simulink library "EOIRParametricModelBlock"  (R2018b)
settings: Solver=VariableStepAuto  StartTime=0.0  StopTime=10.0  RelTol=1e-3
undefined symbols (not defined in the file): ac1dyn_alt0_ft, ac1dyn_lat0_rad, ac1dyn_lon0_rad, ac1IntEOIR_az_bias_rad, ac1IntEOIR_az_random_stddev_rad, ac1IntEOIR_az_tau_s, ac1IntEOIR_azdot_bias_radps, ac1IntEOIR_azdot_random_stddev_radps, ac1IntEOIR_azdot_tau_s, ac1IntEOIR_dt_s, ac1IntEOIR_el_bias_rad, ac1IntEOIR_el_random_stddev_rad, ac1IntEOIR_el_tau_s, ac1IntEOIR_eldot_bias_radps, ac1IntEOIR_eldot_random_stddev_radps, ac1IntEOIR_eldot_tau_s, ac1IntEOIR_range_clrd_noise_flag, ac1IntEOIR_reported_errorCovRAE, ac1IntEOIR_rng_bias_ft, ac1IntEOIR_rng_bias_switch, ac1IntEOIR_rng_random_stddev_ft, ac1IntEOIR_rng_std_dev_gain, ac1IntEOIR_rng_tau_s, ac1IntEOIR_rngdot_bias_ftps, ac1IntEOIR_rngdot_delay_s, ac1IntEOIR_rngdot_random_stddev_ftps, ac1IntEOIR_rngdot_std_dev_gain, ac1IntEOIR_rngdot_tau_s, ac1IntEOIR_seed1, ac1IntEOIR_seed2, ac1IntEOIR_seed3, ac1IntEOIR_seed4, ac1IntEOIR_seed5, ac1IntEOIR_seed6, ac1IntEOIR_sns_for_azimuth_deg, ac1IntEOIR_sns_for_elevation_deg, ac1IntEOIR_sns_max_range_ft
libraries: simulink x11, cart2sph_degas x1, ExtractCovDiag x1, sph2cart x1
settings Model: Creator=BI28030  LastModifiedBy=BI28030
settings SFSimCC: SimUseLocalCustomCode=off
settings RTWCC: RTWUseLocalCustomCode=off
settings CodeAppCC: StateflowObjectComments=on

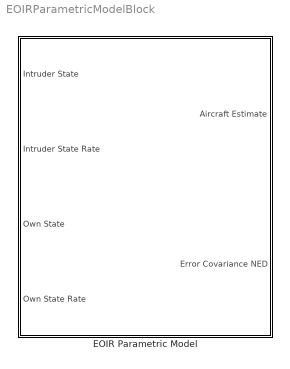
== system EOIRParametricModelBlock ==
  EOIR Parametric Model : Subsystem  mask(EOIR Parametric Model){dt_s=ac1IntEOIR_dt_s, lat0_rad=ac1dyn_lat0_rad, lon0_rad=ac1dyn_lon0_rad, alt0_ft=ac1dyn_alt0_ft, sns_max_range_ft=ac1IntEOIR_sns_max_range_ft, sns_for_azimuth_deg=ac1IntEOIR_sns_for_azimuth_deg, sns_for_elevation_deg=ac1IntEOIR_sns_for_elevation_deg, rng_random_stddev_ft=ac1IntEOIR_rng_random_stddev_ft, rng_bias_ft=ac1IntEOIR_rng_bias_ft, rng_tau_s=ac1IntEOIR_rng_tau_s, seed1=ac1IntEOIR_seed1, rng_std_dev_gain=ac1IntEOIR_rng_std_dev_gain, rng_bias_switch=ac1IntEOIR_rng_bias_switch, coloredNoiseFlag=ac1IntEOIR_range_clrd_noise_flag, az_random_stddev_rad=ac1IntEOIR_az_random_stddev_rad, az_bias_rad=ac1IntEOIR_az_bias_rad, az_tau_s=ac1IntEOIR_az_tau_s, seed2=ac1IntEOIR_seed2, el_random_stddev_rad=ac1IntEOIR_el_random_stddev_rad, el_bias_rad=ac1IntEOIR_el_bias_rad, el_tau_s=ac1IntEOIR_el_tau_s, seed3=ac1IntEOIR_seed3, rngdot_random_stddev_ftps=ac1IntEOIR_rngdot_random_stddev_ftps, rngdot_bias_ftps=ac1IntEOIR_rngdot_bias_ftps, rngdot_tau_s=ac1IntEOIR_rngdot_tau_s, seed4=ac1IntEOIR_seed4, rngdot_std_dev_gain=ac1IntEOIR_rngdot_std_dev_gain, rngdot_delay_s=ac1IntEOIR_rngdot_delay_s, azdot_random_stddev_radps=ac1IntEOIR_azdot_random_stddev_radps, azdot_bias_radps=ac1IntEOIR_azdot_bias_radps, azdot_tau_s=ac1IntEOIR_azdot_tau_s, seed5=ac1IntEOIR_seed5, eldot_random_stddev_radps=ac1IntEOIR_eldot_random_stddev_radps, eldot_bias_radps=ac1IntEOIR_eldot_bias_radps, eldot_tau_s=ac1IntEOIR_eldot_tau_s, seed6=ac1IntEOIR_seed6, covRAE=ac1IntEOIR_reported_errorCovRAE}
      mask prompts: dt_s "Timestep"; lat0_rad "ENU Origin Latitude"; lon0_rad "ENU Origin Longitude"; alt0_ft "ENU Origin Altitude"; sns_max_range_ft "Max Detection Range"; sns_for_azimuth_deg "Field of Regard: Azimuth Limit (deg)"; sns_for_elevation_deg "Field of Regard: Elevation Limit (deg)"; rng_random_stddev_ft "Range Random Error Standard Deviation"; rng_bias_ft "Range Bias"; rng_tau_s "Correlation Time"; seed1 "Random Seed"; rng_std_dev_gain "Standard Deviation gain"; rng_bias_switch "Range Bias Switch"; coloredNoiseFlag "Range Colored Noise Switch"; az_random_stddev_rad "Azimuth Random Error Standard Deviation"; az_bias_rad "Azimuth Bias"; az_tau_s "Correlation Time"; seed2 "Random Seed"; el_random_stddev_rad "Elevation Random Error Standard Deviation"; el_bias_rad "Elevation Bias"; el_tau_s "Correlation Time"; seed3 "Random Seed"; rngdot_random_stddev_ftps "Range Rate Random Error Standard Deviation"; rngdot_bias_ftps "Range Rate Bias"; rngdot_tau_s "Correlation Time"; seed4 "Random Seed"; rngdot_std_dev_gain "Standard Deviation Gain"; rngdot_delay_s "Range-rate Delay time"; azdot_random_stddev_radps "Azimuth Rate Random Error Standrad Deviation"; azdot_bias_radps "Azimuth Rate Bias"; azdot_tau_s "Correlation Time"; seed5 "Random Seed"; eldot_random_stddev_radps "Elevation Rate Random Error Standard Deviation"; eldot_bias_radps "Elevation Rate Bias"; eldot_tau_s "Correlation Time"; seed6 "Random Seed"; covRAE "Error Covariance"
      mask help: Model of an EOIR sensor based off of the RTCA SC-228 EOIR MOPS
      mask Help:
      | Parametric model of an EOIR sensor.  Independent noise is added to
      | each of range, azimuth, elevation and their rates.  Noise is colored using
      | weights determined by time constant parameters.
      | 
      | Output takes the form of a AircraftEstimate data bus and a 6x6 error covariance
      | matrix in North-East-Down.  State order in error covariance output is
      | [ posN posE posD velN velE velD ].
      mask DialogControl ParameterTabVar0 Prompt: Tab
      mask DialogControl ParameterTabVar01 Prompt: Range
      mask DialogControl ParameterTabVar012 Prompt: Azimuth
      mask DialogControl ParameterTabVar0123 Prompt: Elevation
      mask DialogControl ParameterTabVar01234 Prompt: Range rate
      mask DialogControl ParameterTabVar012345 Prompt: Azimuth Rate
      mask DialogControl ParameterTabVar0123456 Prompt: Elevation Rate
      mask DialogControl ParameterTabVar01234567 Prompt: Covariance

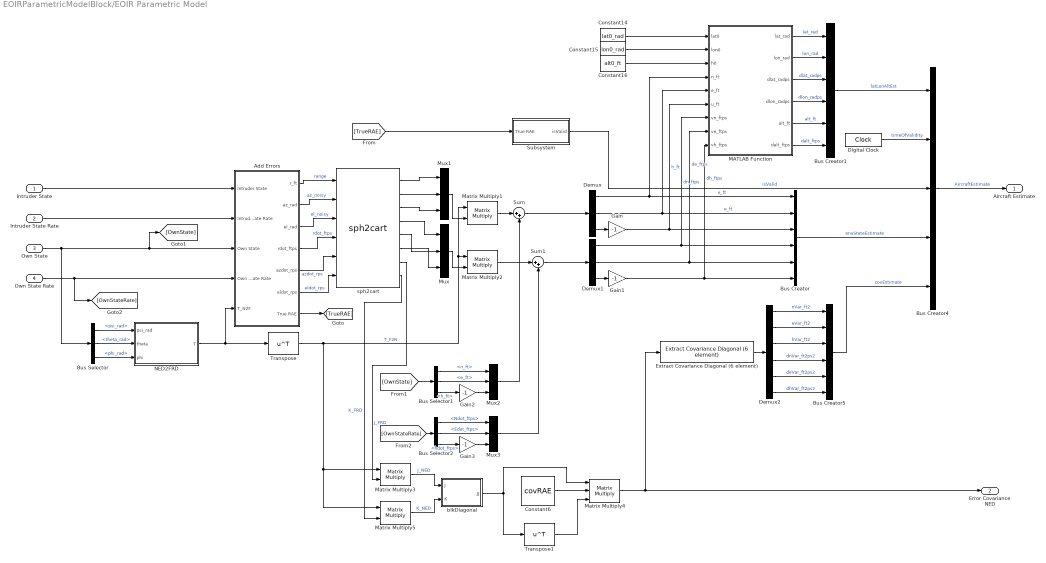
== system EOIRParametricModelBlock/EOIR Parametric Model ==
  Intruder State : Inport  OutDataTypeStr=Bus: AircraftState
  Intruder State Rate : Inport  Port=2  OutDataTypeStr=Bus: AircraftStateRate
  Own State : Inport  Port=3  OutDataTypeStr=Bus: AircraftState
  Own State Rate : Inport  Port=4  OutDataTypeStr=Bus: AircraftStateRate
  Add Errors : Subsystem
  Bus Creator : BusCreator  Inputs=6  OutDataTypeStr=Bus: StateEstimate
  Bus Creator1 : BusCreator  Inputs=6  OutDataTypeStr=Bus: LatLonAltMeasurement
  Bus Creator4 : BusCreator  Inputs='latLonAltEst','timeOfValidity','isValid','enuStateEstimate','covEstimate'  OutDataTypeStr=Bus: AircraftEstimate  NonVirtualBus=on
  Bus Creator5 : BusCreator  Inputs=6  OutDataTypeStr=Bus: CovarianceEstimate
  Bus Selector : BusSelector  OutputSignals=psi_rad,theta_rad,phi_rad
  Bus Selector1 : BusSelector  OutputSignals=n_ft,e_ft,h_ft
  Bus Selector2 : BusSelector  OutputSignals=Ndot_ftps,Edot_ftps,hdot_ftps
  Constant14 : Constant  Value=lat0_rad  OutDataTypeStr=double  SampleTime=dt_s
  Constant15 : Constant  Value=lon0_rad  OutDataTypeStr=double  SampleTime=dt_s
  Constant16 : Constant  Value=alt0_ft  OutDataTypeStr=double  SampleTime=dt_s
  Constant6 : Constant  Value=covRAE
  Demux : Demux  Outputs=3
  Demux1 : Demux  Outputs=3
  Demux2 : Demux  Outputs=6
  Digital Clock : DigitalClock  SampleTime=dt_s
  Extract Covariance Diagonal (6 element) : ExtractCovDiag/Extract Covariance Diagonal (6 element)  SystemSampleTime=-1
  Gain{,1..3} (4 alike) : Gain  Gain=-1
  MATLAB Function : MATLAB Function  TreatAsAtomicUnit=on
  Matrix Multiply{1..3,5} (4 alike) : Product  Multiplication=Matrix(*)
  Matrix Multiply4 : Product  Inputs=3  Multiplication=Matrix(*)
  Mux{,1..3} (4 alike) : Mux  Inputs=3
  NED2FRD : MATLAB Function  TreatAsAtomicUnit=on
  Subsystem : Subsystem
  Sum : Sum  Inputs=|++
  Sum1 : Sum  Inputs=|++
  Transpose : Math  Operator=transpose  SaturateOnIntegerOverflow=on
  Transpose1 : Math  Operator=transpose  SaturateOnIntegerOverflow=on
  blkDiagonal : MATLAB Function  TreatAsAtomicUnit=on
  sph2cart : sph2cart/sph2cart  SystemSampleTime=-1
      settings: SourceProductName=CASSATTv6: Signals Library
  Aircraft Estimate : Outport  OutDataTypeStr=Bus: AircraftEstimate
  Error Covariance NED : Outport  Port=2  OutDataTypeStr=double  PortDimensions=[ 6 6 ]
  wires:
  Add Errors/6(eldot_rps) -> sph2cart/6  "eldot_rps"
  Add Errors/5(azdot_rps) -> sph2cart/5  "azdot_rps"
  Add Errors/4(rdot_ftps) -> sph2cart/4  "rdot_ftps"
  Add Errors/3(el_rad) -> sph2cart/3  "el_noisy"
  Add Errors/2(az_rad) -> sph2cart/2  "az_noisy"
  sph2cart/6 -> Mux/3
  sph2cart/5 -> Mux/2
  sph2cart/4 -> Mux/1
  Matrix Multiply5/1 -> blkDiagonal/2(K)  "K_NED"
  sph2cart/8 -> Matrix Multiply5/2  "K_FRD"
  sph2cart/7 -> Matrix Multiply3/2  "J_FRD"
  Demux/1 -> MATLAB Function/4(n_ft), Bus Creator/1  "n_ft"
  Bus Creator4/1 -> Aircraft Estimate/1  "AircraftEstimate"
  Bus Selector/3 -> NED2FRD/3(phi)  "<phi_rad>"
  Own State/1 -> [OwnState], Add Errors/3(Own State), Bus Selector/1
  Bus Selector/1 -> NED2FRD/1(psi_rad)  "<psi_rad>"
  Bus Selector/2 -> NED2FRD/2(theta)  "<theta_rad>"
  Intruder State/1 -> Add Errors/1(Intruder State)
  Bus Creator5/1 -> Bus Creator4/5  "covEstimate"
  MATLAB Function/6(dalt_ftps) -> Bus Creator1/6  "dalt_ftps"
  MATLAB Function/5(alt_ft) -> Bus Creator1/5  "alt_ft"
  MATLAB Function/4(dlon_radps) -> Bus Creator1/4  "dlon_radps"
  MATLAB Function/3(dlat_radps) -> Bus Creator1/3  "dlat_radps"
  MATLAB Function/2(lon_rad) -> Bus Creator1/2  "lon_rad"
  MATLAB Function/1(lat_rad) -> Bus Creator1/1  "lat_rad"
  Bus Creator1/1 -> Bus Creator4/1  "latLonAltEst"
  Subsystem/1(isValid) -> Bus Creator4/3  "isValid"
  Digital Clock/1 -> Bus Creator4/2  "timeOfValidity"
  Constant14/1 -> MATLAB Function/1(lat0)
  Constant16/1 -> MATLAB Function/3(h0)
  Constant15/1 -> MATLAB Function/2(lon0)
  Bus Creator/1 -> Bus Creator4/4  "enuStateEstimate"
  Gain/1 -> MATLAB Function/6(u_ft), Bus Creator/3  "h_ft"
  Gain1/1 -> MATLAB Function/9(vh_ftps), Bus Creator/6  "dh_ftps"
  Demux1/1 -> MATLAB Function/7(vn_ftps), Bus Creator/4  "dn_ftps"
  Demux1/2 -> MATLAB Function/8(ve_ftps), Bus Creator/5  "de_ftps"
  Transpose/1 -> Matrix Multiply5/1, Matrix Multiply3/1, Matrix Multiply2/1, Matrix Multiply1/1  "T_F2N"
  Add Errors/1(r_ft) -> sph2cart/1  "range"
  NED2FRD/1(T) -> Add Errors/5(T_N2F), Transpose/1
  sph2cart/1 -> Mux1/1
  sph2cart/2 -> Mux1/2
  sph2cart/3 -> Mux1/3
  Mux1/1 -> Matrix Multiply1/2
  Mux/1 -> Matrix Multiply2/2
  Matrix Multiply1/1 -> Sum/1
  Matrix Multiply2/1 -> Sum1/1
  Bus Selector1/1 -> Mux2/1  "<n_ft>"
  Bus Selector1/3 -> Gain2/1  "<h_ft>"
  Bus Selector1/2 -> Mux2/2  "<e_ft>"
  Gain2/1 -> Mux2/3
  Mux2/1 -> Sum/2
  Intruder State Rate/1 -> Add Errors/2(Intruder State Rate)
  Own State Rate/1 -> [OwnStateRate], Add Errors/4(Own State Rate)
  Bus Selector2/3 -> Gain3/1  "<hdot_ftps>"
  Bus Selector2/1 -> Mux3/1  "<Ndot_ftps>"
  Bus Selector2/2 -> Mux3/2  "<Edot_ftps>"
  Gain3/1 -> Mux3/3
  Mux3/1 -> Sum1/2
  Demux/2 -> MATLAB Function/5(e_ft), Bus Creator/2  "e_ft"
  Demux/3 -> Gain/1
  Sum/1 -> Demux/1
  Demux1/3 -> Gain1/1
  Sum1/1 -> Demux1/1
  Matrix Multiply3/1 -> blkDiagonal/1(J)  "J_NED"
  Transpose1/1 -> Matrix Multiply4/3
  Constant6/1 -> Matrix Multiply4/2
  blkDiagonal/1(JJ) -> Transpose1/1, Matrix Multiply4/1
  Matrix Multiply4/1 -> Extract Covariance Diagonal (6 element)/1, Error Covariance NED/1
  Demux2/3 -> Bus Creator5/3  "hVar_ft2"
  Demux2/6 -> Bus Creator5/6  "dhVar_ft2ps2"
  Demux2/4 -> Bus Creator5/4  "dnVar_ft2ps2"
  Demux2/5 -> Bus Creator5/5  "deVar_ft2ps2"
  Demux2/2 -> Bus Creator5/2  "eVar_ft2"
  Demux2/1 -> Bus Creator5/1  "nVar_ft2"
  Add Errors/7(True RAE) -> [TrueRAE]
  [TrueRAE] -> Subsystem/1(True RAE)
  [OwnState] -> Bus Selector1/1
  [OwnStateRate] -> Bus Selector2/1
  Extract Covariance Diagonal (6 element)/1 -> Demux2/1

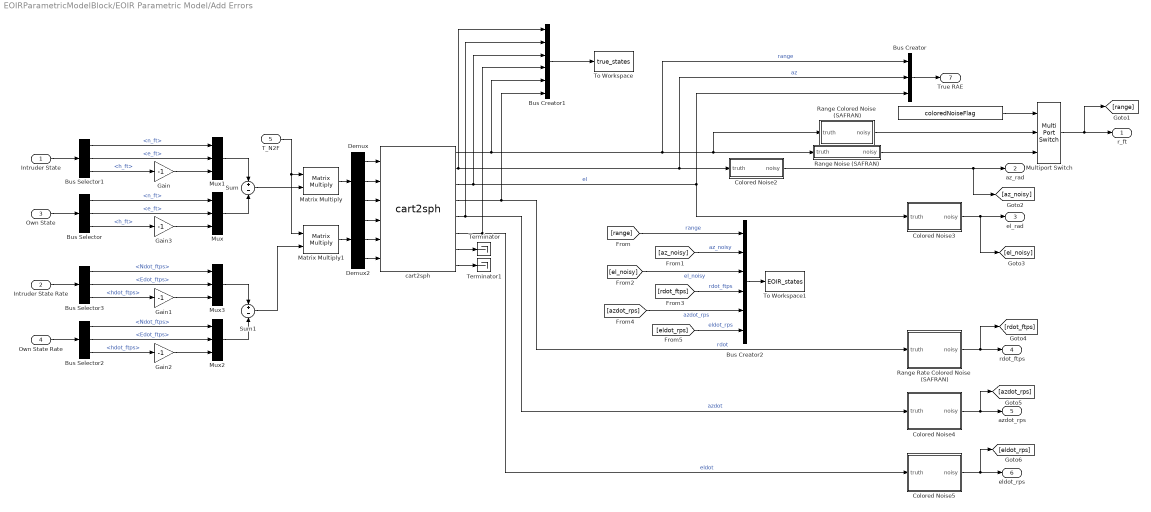
== system EOIRParametricModelBlock/EOIR Parametric Model/Add Errors ==
  Intruder State : Inport  OutDataTypeStr=Bus: AircraftState
  Intruder State Rate : Inport  Port=2  OutDataTypeStr=Bus: AircraftStateRate
  Own State : Inport  Port=3  OutDataTypeStr=Bus: AircraftState
  Own State Rate : Inport  Port=4  OutDataTypeStr=Bus: AircraftStateRate
  T_N2F : Inport  Port=5
  " " : Constant  Value=coloredNoiseFlag
  Bus Creator1 : BusCreator  Inputs=6
  Bus Creator2 : BusCreator  Inputs=6
  Bus Creator : BusCreator  Inputs=3
  Bus Selector : BusSelector  OutputSignals=n_ft,e_ft,h_ft
  Bus Selector1 : BusSelector  OutputSignals=n_ft,e_ft,h_ft
  Bus Selector2 : BusSelector  OutputSignals=Ndot_ftps,Edot_ftps,hdot_ftps
  Bus Selector3 : BusSelector  OutputSignals=Ndot_ftps,Edot_ftps,hdot_ftps
  Colored Noise2 : Subsystem  mask(Colored Noise){sig=az_random_stddev_rad, bias=az_bias_rad, tau=az_tau_s, dt=dt_s, seed=seed2}
      mask prompts: sig "Random error standard deviation"; bias "Bias error"; tau "Correlation time"; dt "Track update time"; seed "Random Seed"
      mask help: Generates a noisy state variable estimate using the ABSAA colored noise model. Set correlation time to zero for white noise.
      mask Help:
      | Generates a noisy state variable estimate using the AF Common ABSAA error
      | model.  Time correlation of the error is defined by an exponential decay
      | of K = exp(-tau/dt), where tau is the correlation time and dt is the time
      | between track updates.  The track error at time t is then:
      | 
      |     err(t) = K*err(t-1) + N(0,(1-K^2)*sig^2) + bias
      | 
      | where N(x,y) is a Gaussian noise process with mean x and variance y and
      | with random number generator seeded with the integer 'seed'.
      | 
      | The random noise process must be initialized with an error drawn from
      | N(0,sig^2).
      | 
      | The noise model can be used to produce white noise by setting tau to zero.
  Colored Noise3 : Subsystem  mask(Colored Noise){sig=el_random_stddev_rad, bias=el_bias_rad, tau=el_tau_s, dt=dt_s, seed=seed3}
      mask prompts: sig "Random error standard deviation"; bias "Bias error"; tau "Correlation time"; dt "Track update time"; seed "Random Seed"
      mask help: Generates a noisy state variable estimate using the ABSAA colored noise model. Set correlation time to zero for white noise.
      mask Help:
      | Generates a noisy state variable estimate using the AF Common ABSAA error
      | model.  Time correlation of the error is defined by an exponential decay
      | of K = exp(-tau/dt), where tau is the correlation time and dt is the time
      | between track updates.  The track error at time t is then:
      | 
      |     err(t) = K*err(t-1) + N(0,(1-K^2)*sig^2) + bias
      | 
      | where N(x,y) is a Gaussian noise process with mean x and variance y and
      | with random number generator seeded with the integer 'seed'.
      | 
      | The random noise process must be initialized with an error drawn from
      | N(0,sig^2).
      | 
      | The noise model can be used to produce white noise by setting tau to zero.
  Colored Noise4 : Subsystem  mask(Colored Noise){sig=azdot_random_stddev_radps, bias=azdot_bias_radps, tau=azdot_tau_s, dt=dt_s, seed=seed5}
      mask prompts: sig "Random error standard deviation"; bias "Bias error"; tau "Correlation time"; dt "Track update time"; seed "Random Seed"
      mask help: Generates a noisy state variable estimate using the ABSAA colored noise model. Set correlation time to zero for white noise.
      mask Help:
      | Generates a noisy state variable estimate using the AF Common ABSAA error
      | model.  Time correlation of the error is defined by an exponential decay
      | of K = exp(-tau/dt), where tau is the correlation time and dt is the time
      | between track updates.  The track error at time t is then:
      | 
      |     err(t) = K*err(t-1) + N(0,(1-K^2)*sig^2) + bias
      | 
      | where N(x,y) is a Gaussian noise process with mean x and variance y and
      | with random number generator seeded with the integer 'seed'.
      | 
      | The random noise process must be initialized with an error drawn from
      | N(0,sig^2).
      | 
      | The noise model can be used to produce white noise by setting tau to zero.
  Colored Noise5 : Subsystem  mask(Colored Noise){sig=eldot_random_stddev_radps, bias=eldot_bias_radps, tau=eldot_tau_s, dt=dt_s, seed=seed6}
      mask prompts: sig "Random error standard deviation"; bias "Bias error"; tau "Correlation time"; dt "Track update time"; seed "Random Seed"
      mask help: Generates a noisy state variable estimate using the ABSAA colored noise model. Set correlation time to zero for white noise.
      mask Help:
      | Generates a noisy state variable estimate using the AF Common ABSAA error
      | model.  Time correlation of the error is defined by an exponential decay
      | of K = exp(-tau/dt), where tau is the correlation time and dt is the time
      | between track updates.  The track error at time t is then:
      | 
      |     err(t) = K*err(t-1) + N(0,(1-K^2)*sig^2) + bias
      | 
      | where N(x,y) is a Gaussian noise process with mean x and variance y and
      | with random number generator seeded with the integer 'seed'.
      | 
      | The random noise process must be initialized with an error drawn from
      | N(0,sig^2).
      | 
      | The noise model can be used to produce white noise by setting tau to zero.
  Demux : Demux  Outputs=3
  Demux2 : Demux  Outputs=3
  Gain{,1..3} (4 alike) : Gain  Gain=-1
  Matrix Multiply : Product  Multiplication=Matrix(*)
  Matrix Multiply1 : Product  Multiplication=Matrix(*)
  Multiport Switch : MultiPortSwitch  DataPortOrder=Specify indices  DataPortIndices={1, 0}
  Mux{,1..3} (4 alike) : Mux  Inputs=3
  Range Colored Noise (SAFRAN) : Subsystem  mask(Colored Noise){sig=rng_random_stddev_ft, bias=rng_bias_ft, tau=rng_tau_s, dt=dt_s, seed=seed1, std_dev_gain=rng_std_dev_gain, range_bias_switch=rng_bias_switch}
      mask prompts: sig "Random error standard deviation"; bias "Bias error"; tau "Correlation time"; dt "Track update time"; seed "Random Seed"; std_dev_gain "Range Standard Deviation Gain"; range_bias_switch "Range Bias Switch"
      mask help: Generates a noisy state variable estimate using the ABSAA colored noise model. Set correlation time to zero for white noise.
      mask Help:
      | Generates a noisy state variable estimate using the AF Common ABSAA error
      | model.  Time correlation of the error is defined by an exponential decay
      | of K = exp(-tau/dt), where tau is the correlation time and dt is the time
      | between track updates.  The track error at time t is then:
      | 
      |     err(t) = K*err(t-1) + N(0,(1-K^2)*sig^2) + bias
      | 
      | where N(x,y) is a Gaussian noise process with mean x and variance y and
      | with random number generator seeded with the integer 'seed'.
      | 
      | The random noise process must be initialized with an error drawn from
      | N(0,sig^2).
      | 
      | The noise model can be used to produce white noise by setting tau to zero.
  Range Noise (SAFRAN) : Subsystem  mask{dt_s=dt_s, seed=seed1}
      mask prompts: dt_s "Track Update Time"; seed "Random Seed"
  Range Rate Colored Noise (SAFRAN) : Subsystem  mask(Colored Noise){sig=rngdot_random_stddev_ftps, bias=rngdot_bias_ftps, tau=rngdot_tau_s, dt=dt_s, seed=seed4, std_dev_gain=rngdot_std_dev_gain}
      mask prompts: sig "Random error standard deviation"; bias "Bias error"; tau "Correlation time"; dt "Track update time"; seed "Random Seed"; std_dev_gain "Standard Deviaton Gain"
      mask help: Generates a noisy state variable estimate using the ABSAA colored noise model. Set correlation time to zero for white noise.
      mask Help:
      | Generates a noisy state variable estimate using the AF Common ABSAA error
      | model.  Time correlation of the error is defined by an exponential decay
      | of K = exp(-tau/dt), where tau is the correlation time and dt is the time
      | between track updates.  The track error at time t is then:
      | 
      |     err(t) = K*err(t-1) + N(0,(1-K^2)*sig^2) + bias
      | 
      | where N(x,y) is a Gaussian noise process with mean x and variance y and
      | with random number generator seeded with the integer 'seed'.
      | 
      | The random noise process must be initialized with an error drawn from
      | N(0,sig^2).
      | 
      | The noise model can be used to produce white noise by setting tau to zero.
  Sum : Sum  Inputs=+-
  Sum1 : Sum  Inputs=+-
  Terminator : Terminator
  Terminator1 : Terminator
  To Workspace : ToWorkspace  VariableName=true_states  SaveFormat=Timeseries  SampleTime=-1
  To Workspace1 : ToWorkspace  VariableName=EOIR_states  SaveFormat=Timeseries  SampleTime=-1
  cart2sph : cart2sph_degas/cart2sph  SystemSampleTime=-1
  r_ft : Outport
  az_rad : Outport  Port=2
  el_rad : Outport  Port=3
  rdot_ftps : Outport  Port=4
  azdot_rps : Outport  Port=5
  eldot_rps : Outport  Port=6
  True RAE : Outport  Port=7
  wires:
  Range Rate Colored Noise (SAFRAN)/1(noisy) -> [rdot_ftps], rdot_ftps/1
  cart2sph/8 -> Terminator1/1
  cart2sph/7 -> Terminator/1
  Demux2/3 -> cart2sph/6
  Demux2/2 -> cart2sph/5
  Demux2/1 -> cart2sph/4
  cart2sph/4 -> Range Rate Colored Noise (SAFRAN)/1(truth), Bus Creator1/6  "rdot"
  Matrix Multiply1/1 -> Demux2/1
  Demux/1 -> cart2sph/1
  Demux/2 -> cart2sph/2
  Demux/3 -> cart2sph/3
  Matrix Multiply/1 -> Demux/1
  Sum1/1 -> Matrix Multiply1/2
  Sum/1 -> Matrix Multiply/2
  T_N2F/1 -> Matrix Multiply/1, Matrix Multiply1/1
  Gain3/1 -> Mux/3
  Gain/1 -> Mux1/3
  Gain2/1 -> Mux2/3
  Gain1/1 -> Mux3/3
  Mux2/1 -> Sum1/2
  Mux3/1 -> Sum1/1
  Bus Selector2/2 -> Mux2/2  "<Edot_ftps>"
  Bus Selector2/1 -> Mux2/1  "<Ndot_ftps>"
  Bus Selector2/3 -> Gain2/1  "<hdot_ftps>"
  Own State Rate/1 -> Bus Selector2/1
  Intruder State Rate/1 -> Bus Selector3/1
  Bus Selector3/2 -> Mux3/2  "<Edot_ftps>"
  Bus Selector3/1 -> Mux3/1  "<Ndot_ftps>"
  Bus Selector3/3 -> Gain1/1  "<hdot_ftps>"
  Mux/1 -> Sum/2
  Mux1/1 -> Sum/1
  Intruder State/1 -> Bus Selector1/1
  Bus Selector1/2 -> Mux1/2  "<e_ft>"
  Bus Selector1/1 -> Mux1/1  "<n_ft>"
  Bus Selector1/3 -> Gain/1  "<h_ft>"
  Bus Selector/2 -> Mux/2  "<e_ft>"
  Bus Selector/1 -> Mux/1  "<n_ft>"
  Bus Selector/3 -> Gain3/1  "<h_ft>"
  Own State/1 -> Bus Selector/1
  cart2sph/1 -> Range Colored Noise (SAFRAN)/1(truth), Range Noise (SAFRAN)/1(truth), Bus Creator/1, Bus Creator1/5  "range"
  cart2sph/2 -> Colored Noise2/1(truth), Bus Creator/2, Bus Creator1/1  "az"
  cart2sph/3 -> Bus Creator/3, Colored Noise3/1(truth), Bus Creator1/3  "el"
  cart2sph/5 -> Colored Noise4/1(truth), Bus Creator1/2  "azdot"
  cart2sph/6 -> Colored Noise5/1(truth), Bus Creator1/4  "eldot"
  Colored Noise2/1(noisy) -> [az_noisy], az_rad/1
  Colored Noise3/1(noisy) -> [el_noisy], el_rad/1
  Colored Noise4/1(noisy) -> [azdot_rps], azdot_rps/1
  Colored Noise5/1(noisy) -> [eldot_rps], eldot_rps/1
  Bus Creator/1 -> True RAE/1
  Range Colored Noise (SAFRAN)/1(noisy) -> Multiport Switch/2
  Bus Creator1/1 -> To Workspace/1
  Multiport Switch/1 -> [range], r_ft/1
  Range Noise (SAFRAN)/1(noisy) -> Multiport Switch/3
  " "/1 -> Multiport Switch/1
  [range] -> Bus Creator2/1  "range"
  [azdot_rps] -> Bus Creator2/5  "azdot_rps"
  Bus Creator2/1 -> To Workspace1/1
  [el_noisy] -> Bus Creator2/3  "el_noisy"
  [az_noisy] -> Bus Creator2/2  "az_noisy"
  [rdot_ftps] -> Bus Creator2/4  "rdot_ftps"
  [eldot_rps] -> Bus Creator2/6  "eldot_rps"

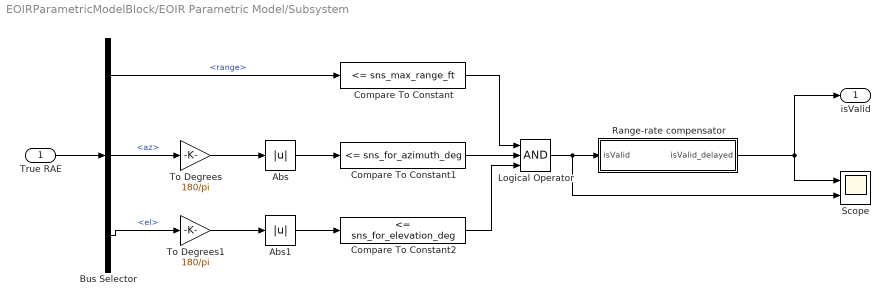
== system EOIRParametricModelBlock/EOIR Parametric Model/Subsystem ==
  True RAE : Inport
  Abs : Abs
  Abs1 : Abs
  Bus Selector : BusSelector  OutputSignals=range,az,el
  Compare To Constant : simulink/Logic and Bit Operations/Compare To Constant  relop=<=  const=sns_max_range_ft  OutDataTypeStr=boolean
  Compare To Constant1 : simulink/Logic and Bit Operations/Compare To Constant  relop=<=  const=sns_for_azimuth_deg  OutDataTypeStr=boolean
  Compare To Constant2 : simulink/Logic and Bit Operations/Compare To Constant  relop=<=  const=sns_for_elevation_deg  OutDataTypeStr=boolean
  Logical Operator : Logic  Inputs=3  AllPortsSameDT=off  OutDataTypeStr=boolean
  Range-rate compensator : Subsystem
  Scope : Scope  NumInputPorts=2
  To Degrees : Gain  Gain=180/pi
  To Degrees1 : Gain  Gain=180/pi
  isValid : Outport
  wires:
  Range-rate compensator/1(isValid_delayed) -> isValid/1, Scope/1
  True RAE/1 -> Bus Selector/1
  Bus Selector/1 -> Compare To Constant/1  "<range>"
  Logical Operator/1 -> Scope/2, Range-rate compensator/1(isValid)
  Compare To Constant/1 -> Logical Operator/1
  Abs/1 -> Compare To Constant1/1
  Bus Selector/2 -> To Degrees/1  "<az>"
  Bus Selector/3 -> To Degrees1/1  "<el>"
  Abs1/1 -> Compare To Constant2/1
  Compare To Constant1/1 -> Logical Operator/2
  Compare To Constant2/1 -> Logical Operator/3
  To Degrees/1 -> Abs/1
  To Degrees1/1 -> Abs1/1

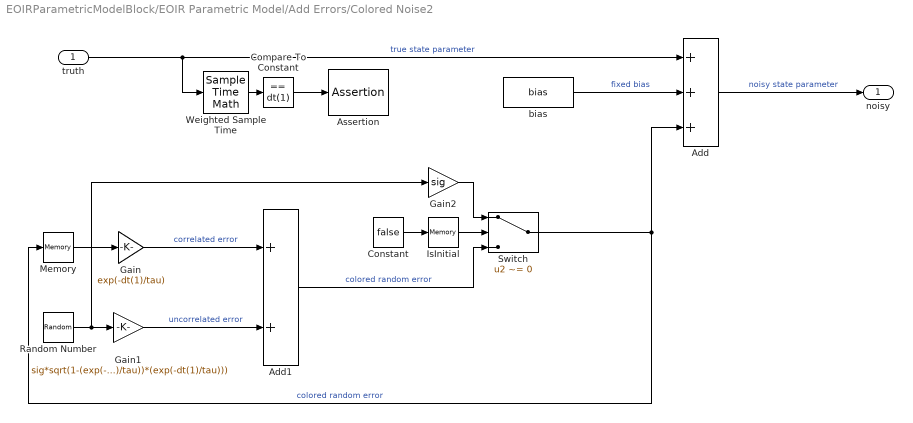
== system EOIRParametricModelBlock/EOIR Parametric Model/Add Errors/Colored Noise2 ==
  truth : Inport
  Add : Sum  Inputs=+++  SampleTime=dt
  Add1 : Sum  SampleTime=dt
  Assertion : Assertion
  Compare To Constant : simulink/Logic and Bit Operations/Compare To Constant  relop===  const=dt(1)  OutDataTypeStr=boolean
  Constant : Constant  Value=false
  Gain : Gain  Gain=exp(-dt(1)/tau)  SampleTime=dt
  Gain1 : Gain  Gain=sig*sqrt(1-(exp(-dt(1)/tau))*(exp(-dt(1)/tau)))
  Gain2 : Gain  Gain=sig
  IsInitial : Memory  InitialCondition=true  InheritSampleTime=on
  Memory : Memory  InheritSampleTime=on
  Random Number : RandomNumber  Seed=seed  SampleTime=dt_s
  Switch : Switch  Criteria=u2 ~= 0  SampleTime=dt
  Weighted Sample Time : SampleTimeMath  TsampMathOp=Ts Only
  bias : Constant  Value=bias
  noisy : Outport
  wires:
  Gain1/1 -> Add1/2  "uncorrelated error"
  Switch/1 -> Memory/1, Add/3  "colored random error"
  bias/1 -> Add/2  "fixed bias"
  Random Number/1 -> Gain2/1, Gain1/1
  Gain/1 -> Add1/1  "correlated error"
  Add/1 -> noisy/1  "noisy state parameter"
  truth/1 -> Weighted Sample Time/1, Add/1  "true state parameter"
  Memory/1 -> Gain/1
  Constant/1 -> IsInitial/1
  IsInitial/1 -> Switch/2
  Add1/1 -> Switch/3  "colored random error"
  Gain2/1 -> Switch/1
  Weighted Sample Time/1 -> Compare To Constant/1
  Compare To Constant/1 -> Assertion/1

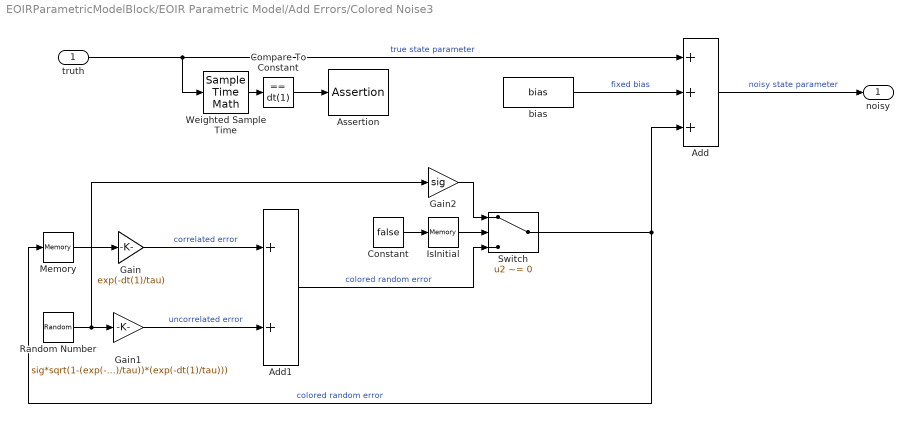
== system EOIRParametricModelBlock/EOIR Parametric Model/Add Errors/Colored Noise3 ==
  truth : Inport
  Add : Sum  Inputs=+++  SampleTime=dt
  Add1 : Sum  SampleTime=dt
  Assertion : Assertion
  Compare To Constant : simulink/Logic and Bit Operations/Compare To Constant  relop===  const=dt(1)  OutDataTypeStr=boolean
  Constant : Constant  Value=false
  Gain : Gain  Gain=exp(-dt(1)/tau)  SampleTime=dt
  Gain1 : Gain  Gain=sig*sqrt(1-(exp(-dt(1)/tau))*(exp(-dt(1)/tau)))
  Gain2 : Gain  Gain=sig
  IsInitial : Memory  InitialCondition=true  InheritSampleTime=on
  Memory : Memory  InheritSampleTime=on
  Random Number : RandomNumber  Seed=seed  SampleTime=dt_s
  Switch : Switch  Criteria=u2 ~= 0  SampleTime=dt
  Weighted Sample Time : SampleTimeMath  TsampMathOp=Ts Only
  bias : Constant  Value=bias
  noisy : Outport
  wires:
  Gain1/1 -> Add1/2  "uncorrelated error"
  Switch/1 -> Memory/1, Add/3  "colored random error"
  bias/1 -> Add/2  "fixed bias"
  Random Number/1 -> Gain2/1, Gain1/1
  Gain/1 -> Add1/1  "correlated error"
  Add/1 -> noisy/1  "noisy state parameter"
  truth/1 -> Weighted Sample Time/1, Add/1  "true state parameter"
  Memory/1 -> Gain/1
  Constant/1 -> IsInitial/1
  IsInitial/1 -> Switch/2
  Add1/1 -> Switch/3  "colored random error"
  Gain2/1 -> Switch/1
  Weighted Sample Time/1 -> Compare To Constant/1
  Compare To Constant/1 -> Assertion/1

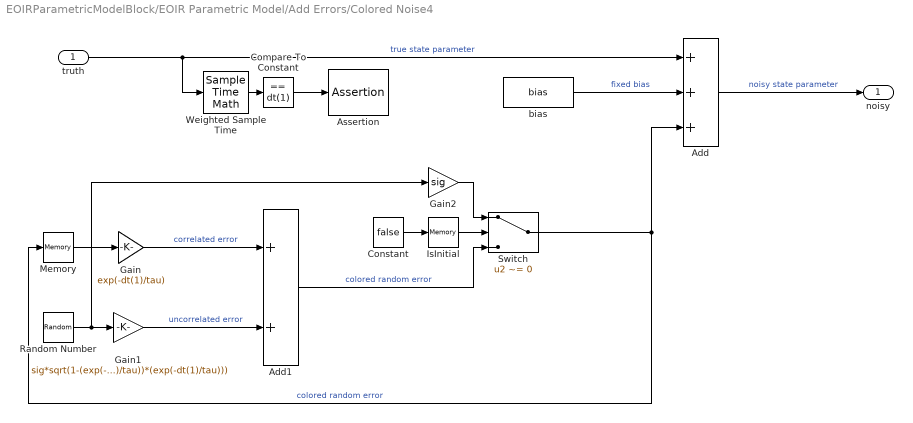
== system EOIRParametricModelBlock/EOIR Parametric Model/Add Errors/Colored Noise4 ==
  truth : Inport
  Add : Sum  Inputs=+++  SampleTime=dt
  Add1 : Sum  SampleTime=dt
  Assertion : Assertion
  Compare To Constant : simulink/Logic and Bit Operations/Compare To Constant  relop===  const=dt(1)  OutDataTypeStr=boolean
  Constant : Constant  Value=false
  Gain : Gain  Gain=exp(-dt(1)/tau)  SampleTime=dt
  Gain1 : Gain  Gain=sig*sqrt(1-(exp(-dt(1)/tau))*(exp(-dt(1)/tau)))
  Gain2 : Gain  Gain=sig
  IsInitial : Memory  InitialCondition=true  InheritSampleTime=on
  Memory : Memory  InheritSampleTime=on
  Random Number : RandomNumber  Seed=seed  SampleTime=dt_s
  Switch : Switch  Criteria=u2 ~= 0  SampleTime=dt
  Weighted Sample Time : SampleTimeMath  TsampMathOp=Ts Only
  bias : Constant  Value=bias
  noisy : Outport
  wires:
  Gain1/1 -> Add1/2  "uncorrelated error"
  Switch/1 -> Memory/1, Add/3  "colored random error"
  bias/1 -> Add/2  "fixed bias"
  Random Number/1 -> Gain2/1, Gain1/1
  Gain/1 -> Add1/1  "correlated error"
  Add/1 -> noisy/1  "noisy state parameter"
  truth/1 -> Weighted Sample Time/1, Add/1  "true state parameter"
  Memory/1 -> Gain/1
  Constant/1 -> IsInitial/1
  IsInitial/1 -> Switch/2
  Add1/1 -> Switch/3  "colored random error"
  Gain2/1 -> Switch/1
  Weighted Sample Time/1 -> Compare To Constant/1
  Compare To Constant/1 -> Assertion/1

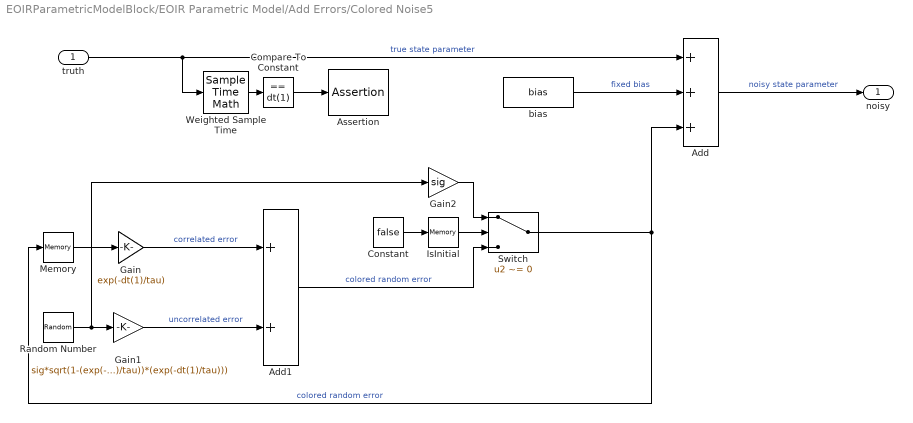
== system EOIRParametricModelBlock/EOIR Parametric Model/Add Errors/Colored Noise5 ==
  truth : Inport
  Add : Sum  Inputs=+++  SampleTime=dt
  Add1 : Sum  SampleTime=dt
  Assertion : Assertion
  Compare To Constant : simulink/Logic and Bit Operations/Compare To Constant  relop===  const=dt(1)  OutDataTypeStr=boolean
  Constant : Constant  Value=false
  Gain : Gain  Gain=exp(-dt(1)/tau)  SampleTime=dt
  Gain1 : Gain  Gain=sig*sqrt(1-(exp(-dt(1)/tau))*(exp(-dt(1)/tau)))
  Gain2 : Gain  Gain=sig
  IsInitial : Memory  InitialCondition=true  InheritSampleTime=on
  Memory : Memory  InheritSampleTime=on
  Random Number : RandomNumber  Seed=seed  SampleTime=dt_s
  Switch : Switch  Criteria=u2 ~= 0  SampleTime=dt
  Weighted Sample Time : SampleTimeMath  TsampMathOp=Ts Only
  bias : Constant  Value=bias
  noisy : Outport
  wires:
  Gain1/1 -> Add1/2  "uncorrelated error"
  Switch/1 -> Memory/1, Add/3  "colored random error"
  bias/1 -> Add/2  "fixed bias"
  Random Number/1 -> Gain2/1, Gain1/1
  Gain/1 -> Add1/1  "correlated error"
  Add/1 -> noisy/1  "noisy state parameter"
  truth/1 -> Weighted Sample Time/1, Add/1  "true state parameter"
  Memory/1 -> Gain/1
  Constant/1 -> IsInitial/1
  IsInitial/1 -> Switch/2
  Add1/1 -> Switch/3  "colored random error"
  Gain2/1 -> Switch/1
  Weighted Sample Time/1 -> Compare To Constant/1
  Compare To Constant/1 -> Assertion/1

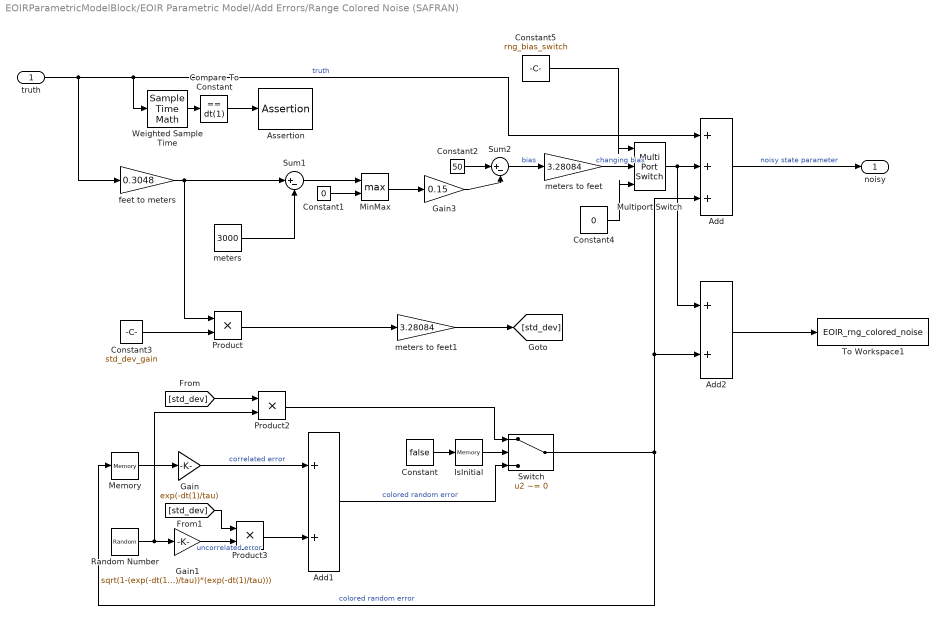
== system EOIRParametricModelBlock/EOIR Parametric Model/Add Errors/Range Colored Noise (SAFRAN) ==
  truth : Inport
  Add : Sum  Inputs=+++  SampleTime=dt
  Add1 : Sum  SampleTime=dt
  Add2 : Sum  SampleTime=dt
  Assertion : Assertion
  Compare To Constant : simulink/Logic and Bit Operations/Compare To Constant  relop===  const=dt(1)  OutDataTypeStr=boolean
  Constant : Constant  Value=false
  Constant1 : Constant  Value=0
  Constant2 : Constant  Value=50
  Constant3 : Constant  Value=std_dev_gain
  Constant4 : Constant  Value=0
  Constant5 : Constant  Value=rng_bias_switch
  Gain : Gain  Gain=exp(-dt(1)/tau)  SampleTime=dt
  Gain1 : Gain  Gain=sqrt(1-(exp(-dt(1)/tau))*(exp(-dt(1)/tau)))
  Gain3 : Gain  Gain=0.15
  IsInitial : Memory  InitialCondition=true  InheritSampleTime=on
  Memory : Memory  InheritSampleTime=on
  MinMax : MinMax  Function=max  Inputs=2
  Multiport Switch : MultiPortSwitch  DataPortOrder=Specify indices  DataPortIndices={1,0}
  Product : Product
  Product2 : Product
  Product3 : Product
  Random Number : RandomNumber  Seed=seed  SampleTime=dt_s
  Sum1 : Sum  Inputs=|+-
  Sum2 : Sum  Inputs=|+-
  Switch : Switch  Criteria=u2 ~= 0  SampleTime=dt
  To Workspace1 : ToWorkspace  VariableName=EOIR_rng_colored_noise  SampleTime=-1
  Weighted Sample Time : SampleTimeMath  TsampMathOp=Ts Only
  feet to meters : Gain  Gain=0.3048
  meters : Constant  Value=3000
  meters to feet : Gain  Gain=3.28084
  meters to feet1 : Gain  Gain=3.28084
  noisy : Outport
  wires:
  Switch/1 -> Memory/1, Add2/2, Add/3  "colored random error"
  Random Number/1 -> Product2/2, Gain1/1
  Gain/1 -> Add1/1  "correlated error"
  Add/1 -> noisy/1  "noisy state parameter"
  Memory/1 -> Gain/1
  Constant/1 -> IsInitial/1
  IsInitial/1 -> Switch/2
  Add1/1 -> Switch/3  "colored random error"
  Product2/1 -> Switch/1
  Weighted Sample Time/1 -> Compare To Constant/1
  Compare To Constant/1 -> Assertion/1
  truth/1 -> Add/1, Weighted Sample Time/1, feet to meters/1  "truth"
  feet to meters/1 -> Product/1, Sum1/1
  meters/1 -> Sum1/2
  Sum1/1 -> MinMax/1
  Constant1/1 -> MinMax/2
  MinMax/1 -> Gain3/1
  Gain3/1 -> Sum2/2
  Constant2/1 -> Sum2/1
  Sum2/1 -> meters to feet/1  "bias"
  Constant3/1 -> Product/2
  Product/1 -> meters to feet1/1
  meters to feet1/1 -> [std_dev]
  [std_dev] -> Product2/1
  Gain1/1 -> Product3/2  "uncorrelated error"
  Product3/1 -> Add1/2
  [std_dev] -> Product3/1
  Add2/1 -> To Workspace1/1
  meters to feet/1 -> Multiport Switch/2  "changing bias"
  Multiport Switch/1 -> Add2/1, Add/2
  Constant4/1 -> Multiport Switch/3
  Constant5/1 -> Multiport Switch/1

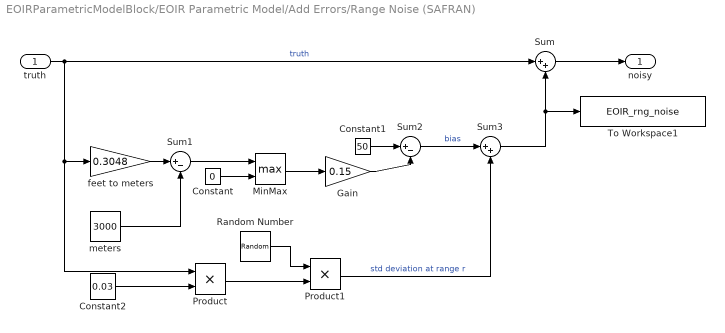
== system EOIRParametricModelBlock/EOIR Parametric Model/Add Errors/Range Noise (SAFRAN) ==
  truth : Inport
  Constant : Constant  Value=0
  Constant1 : Constant  Value=50
  Constant2 : Constant  Value=0.03
  Gain : Gain  Gain=0.15
  MinMax : MinMax  Function=max  Inputs=2
  Product : Product
  Product1 : Product
  Random Number : RandomNumber  Seed=seed  SampleTime=dt_s
  Sum : Sum  Inputs=|++
  Sum1 : Sum  Inputs=|+-
  Sum2 : Sum  Inputs=|+-
  Sum3 : Sum  Inputs=|++
  To Workspace1 : ToWorkspace  VariableName=EOIR_rng_noise  SampleTime=-1
  feet to meters : Gain  Gain=0.3048
  meters : Constant  Value=3000
  noisy : Outport
  wires:
  truth/1 -> Sum/1, feet to meters/1, Product/1  "truth"
  feet to meters/1 -> Sum1/1
  meters/1 -> Sum1/2
  Sum1/1 -> MinMax/1
  Constant/1 -> MinMax/2
  MinMax/1 -> Gain/1
  Gain/1 -> Sum2/2
  Constant1/1 -> Sum2/1
  Sum2/1 -> Sum3/1  "bias"
  Constant2/1 -> Product/2
  Random Number/1 -> Product1/1
  Product/1 -> Product1/2
  Product1/1 -> Sum3/2  "std deviation at range r"
  Sum/1 -> noisy/1
  Sum3/1 -> To Workspace1/1, Sum/2

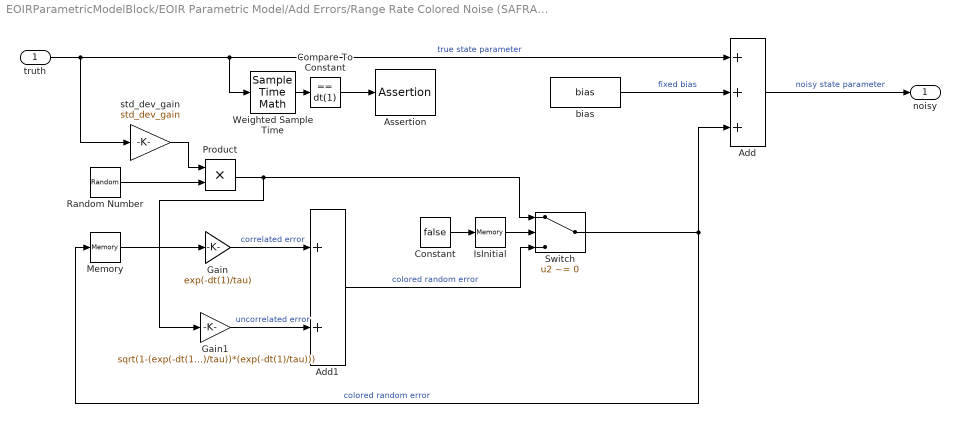
== system EOIRParametricModelBlock/EOIR Parametric Model/Add Errors/Range Rate Colored Noise (SAFRAN) ==
  truth : Inport
  Add : Sum  Inputs=+++  SampleTime=dt
  Add1 : Sum  SampleTime=dt
  Assertion : Assertion
  Compare To Constant : simulink/Logic and Bit Operations/Compare To Constant  relop===  const=dt(1)  OutDataTypeStr=boolean
  Constant : Constant  Value=false
  Gain : Gain  Gain=exp(-dt(1)/tau)  SampleTime=dt
  Gain1 : Gain  Gain=sqrt(1-(exp(-dt(1)/tau))*(exp(-dt(1)/tau)))
  IsInitial : Memory  InitialCondition=true  InheritSampleTime=on
  Memory : Memory  InheritSampleTime=on
  Product : Product
  Random Number : RandomNumber  Seed=seed  SampleTime=dt_s
  Switch : Switch  Criteria=u2 ~= 0  SampleTime=dt
  Weighted Sample Time : SampleTimeMath  TsampMathOp=Ts Only
  bias : Constant  Value=bias
  std_dev_gain : Gain  Gain=std_dev_gain
  noisy : Outport
  wires:
  IsInitial/1 -> Switch/2
  Gain1/1 -> Add1/2  "uncorrelated error"
  Switch/1 -> Memory/1, Add/3  "colored random error"
  bias/1 -> Add/2  "fixed bias"
  Random Number/1 -> Product/2
  Gain/1 -> Add1/1  "correlated error"
  Add/1 -> noisy/1  "noisy state parameter"
  truth/1 -> std_dev_gain/1, Weighted Sample Time/1, Add/1  "true state parameter"
  Memory/1 -> Gain/1
  Constant/1 -> IsInitial/1
  Add1/1 -> Switch/3  "colored random error"
  Weighted Sample Time/1 -> Compare To Constant/1
  Compare To Constant/1 -> Assertion/1
  std_dev_gain/1 -> Product/1
  Product/1 -> Switch/1, Gain1/1

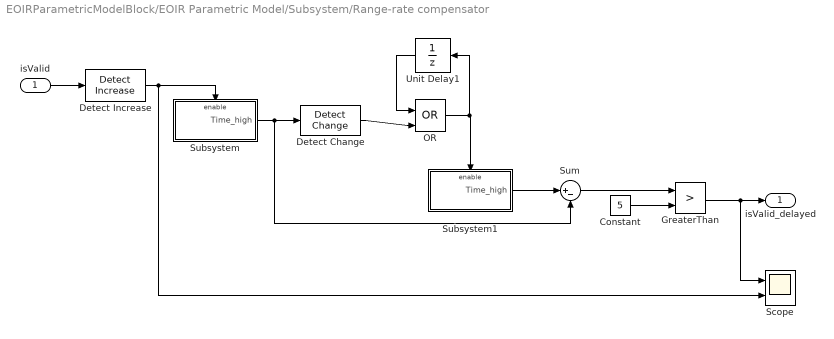
== system EOIRParametricModelBlock/EOIR Parametric Model/Subsystem/Range-rate compensator ==
  isValid : Inport
  Constant : Constant  Value=5
  Detect Change : simulink/Logic and Bit Operations/Detect Change  vinit=0  OutDataTypeStr=boolean
  Detect Increase : simulink/Logic and Bit Operations/Detect Increase  vinit=0.0  OutDataTypeStr=boolean
  GreaterThan : RelationalOperator  Operator=>  OutDataTypeStr=boolean  RndMeth=Simplest
  OR : Logic  Operator=OR  IconShape=distinctive  AllPortsSameDT=off  OutDataTypeStr=boolean
  Scope : Scope  NumInputPorts=2
  Subsystem : Subsystem
  Subsystem1 : Subsystem
  Sum : Sum  Inputs=|+-
  Unit Delay1 : UnitDelay  SampleTime=-1
  isValid_delayed : Outport
  wires:
  isValid/1 -> Detect Increase/1
  Detect Increase/1 -> Scope/2, Subsystem/Enable
  Subsystem/1(Time_high) -> Sum/2, Detect Change/1
  Detect Change/1 -> OR/2
  Unit Delay1/1 -> OR/1
  OR/1 -> Subsystem1/Enable, Unit Delay1/1
  Subsystem1/1(Time_high) -> Sum/1
  Sum/1 -> GreaterThan/1
  Constant/1 -> GreaterThan/2
  GreaterThan/1 -> Scope/1, isValid_delayed/1

== system EOIRParametricModelBlock/EOIR Parametric Model/Subsystem/Range-rate compensator/Subsystem ==
  Enable : EnablePort
  Digital Clock : DigitalClock  SampleTime=.1
  Time_high : Outport  InitialOutput=0
  wires:
  Digital Clock/1 -> Time_high/1

== system EOIRParametricModelBlock/EOIR Parametric Model/Subsystem/Range-rate compensator/Subsystem1 ==
  Enable : EnablePort
  Digital Clock : DigitalClock  SampleTime=.1
  Time_high : Outport  InitialOutput=0
  wires:
  Digital Clock/1 -> Time_high/1

== matlab function EOIRParametricModelBlock/EOIR Parametric Model/MATLAB Function ==
  data: lat0 input double; lon0 input double; h0 input double; n_ft input double; e_ft input double size=1; u_ft input double; vn_ftps input double; ve_ftps input double; vh_ftps input double; lat_rad output double; lon_rad output double; dlat_radps output double; dlon_radps output double; alt_ft output double; dalt_ftps output double
function [lat_rad,lon_rad,dlat_radps,dlon_radps,alt_ft,dalt_ftps] = convertToLLA(lat0,lon0,h0,n_ft,e_ft,u_ft,vn_ftps,ve_ftps,vh_ftps)
%#codegen

% WGS-84 ellipsoid constants
a = 2.09256*10^7;          %Semi-major axis (meters)
f = 1.0/298.257223563;  %Flattening
ecc_sq = f*(2.0-f);        %Eccentricity^2


% Ellipsoidal "radius"
er = a./sqrt(1-ecc_sq.*sin(lat0).^2);


% ECEF coordinates
x0 = (er + h0)*cos(lat0)*cos(lon0);
y0 = (er + h0)*cos(lat0)*sin(lon0);
z0 = (er.*(1-ecc_sq) + h0)*sin(lat0);


%% Rotation Matrix
posECEF0 = [x0;y0;z0];
% Compute the local Up unit vector
vHatU = posECEF0;
vHatU(3) = vHatU(3) ./ ((1-f)^2);
vHatU = vHatU ./ norm(vHatU);

% Compute the projection onto the local Up vector
pU = vHatU * vHatU';

% Compute the projection onto the local Tangent plane
pT = eye(size(pU)) - pU;

% Compute the local North unit vector
vHatZ = [0;0;1];
vHatN = pT * vHatZ;
vHatN = vHatN ./ norm(vHatN);

% Compute the local East unit vector
vHatE = cross(vHatN,vHatU);

% Compute ENU rotation matrix
rotMatENU = zeros(3,3);
rotMatENU(:,1) = vHatE;
rotMatENU(:,2) = vHatN;
rotMatENU(:,3) = vHatU;

tPosECEF = rotMatENU*[e_ft;n_ft;u_ft] + [x0;y0;z0];


%% ECEF to LLA
% WGS-84 derived parameters
b = (1-f).*a;                       %Semi-minor axis (meters)
ecc1_sq = (a.^2 - b.^2)./(a.^2);    %First eccentricity squared
ecc2_sq = (a.^2 - b.^2)./(b.^2);    %Second eccentricity squared


% Length of position vector in equatorial plane
rho = sqrt(tPosECEF(1).^2 + tPosECEF(2).^2);

% Auxillary angle
theta = atan( (tPosECEF(3).*a)./(rho.*b) );

lon_rad = atan2(tPosECEF(2),tPosECEF(1));
lat_rad = atan( (tPosECEF(3) + ecc2_sq.*b.*(sin(theta)).^3)./(rho - ecc1_sq.*a.*(cos(theta)).^3) );

ewRadCurv = a./sqrt(1-ecc1_sq.*sin(lat_rad).^2);

alt_ft = (rho./cos(lat_rad)) - ewRadCurv;


%% Velocities - Project 1 sec into future and use to estimate
dalt_ftps = vh_ftps; % Assume about the same


tPosECEF_1sec = rotMatENU*[e_ft+ve_ftps;...
                           n_ft+vn_ftps;...
                           u_ft] + ...
                           [x0;y0;z0];

% Length of position vector in equatorial plane
rho = sqrt(tPosECEF_1sec(1).^2 + tPosECEF_1sec(2).^2);

% Auxillary angle
theta = atan( (tPosECEF_1sec(3).*a)./(rho.*b) );

lon_rad_1sec = atan2(tPosECEF_1sec(2),tPosECEF_1sec(1));
lat_rad_1sec = atan( (tPosECEF_1sec(3) + ecc2_sq.*b.*(sin(theta)).^3)./(rho - ecc1_sq.*a.*(cos(theta)).^3) );

dlat_radps = lat_rad_1sec - lat_rad;
dlon_radps = lon_rad_1sec - lon_rad;
end

== matlab function EOIRParametricModelBlock/EOIR Parametric Model/NED2FRD ==
  data: psi_rad input; T output; theta input; phi input
function T = Transform_NED2FRD(psi_rad,theta,phi)
%#codegen

yaw = [ cos(psi_rad) sin(psi_rad) 0;
       -sin(psi_rad) cos(psi_rad) 0;
               0        0 1 ];
           
pitch = [ cos(theta) 0 -sin(theta);
                   0 1           0;
          sin(theta) 0  cos(theta) ];
      
roll = [ 1         0        0;
         0  cos(phi) sin(phi);
         0 -sin(phi) cos(phi) ];
     
T = roll*pitch*yaw;     % transformation FROM geographic coord TO body coord

== matlab function EOIRParametricModelBlock/EOIR Parametric Model/blkDiagonal ==
  data: J input double size=[ 3 3 ]; JJ output double size=[ 6 6 ]; K input
function JJ = fcn(J,K)
%#codegen

JJ = [ J zeros(3); K J];
